simulink model "LaneMergingSim_ControllerWithVirtualHuman"  (R2015a)
settings: Solver=ode3  StartTime=0.0  StopTime=11.0  FixedStep=0.1  RelTol=1e-3
libraries: simulink x1
settings Model: Creator=ppnathan  LastModifiedBy=ppnathan

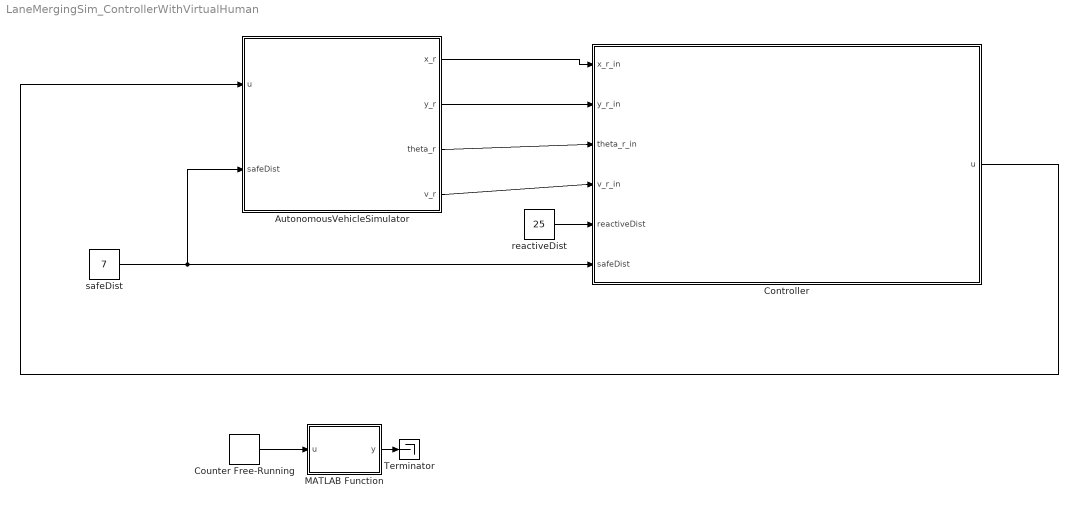
== system LaneMergingSim_ControllerWithVirtualHuman ==
  AutonomousVehicleSimulator : Subsystem
  Controller : Subsystem
  Counter Free-Running : simulink/Sources/Counter Free-Running  NumBits=32  tsamp=-1
  MATLAB Function : MATLAB Function  TreatAsAtomicUnit=on
  Terminator : Terminator
  reactiveDist : Constant  Value=25
  safeDist : Constant  Value=7
  wires:
  AutonomousVehicleSimulator/1(x_r) -> Controller/1(x_r_in)
  AutonomousVehicleSimulator/2(y_r) -> Controller/2(y_r_in)
  AutonomousVehicleSimulator/3(theta_r) -> Controller/3(theta_r_in)
  AutonomousVehicleSimulator/4(v_r) -> Controller/4(v_r_in)
  reactiveDist/1 -> Controller/5(reactiveDist)
  safeDist/1 -> AutonomousVehicleSimulator/2(safeDist), Controller/6(safeDist)
  Controller/1(u) -> AutonomousVehicleSimulator/1(u)
  Counter Free-Running/1 -> MATLAB Function/1(u)
  MATLAB Function/1(y) -> Terminator/1

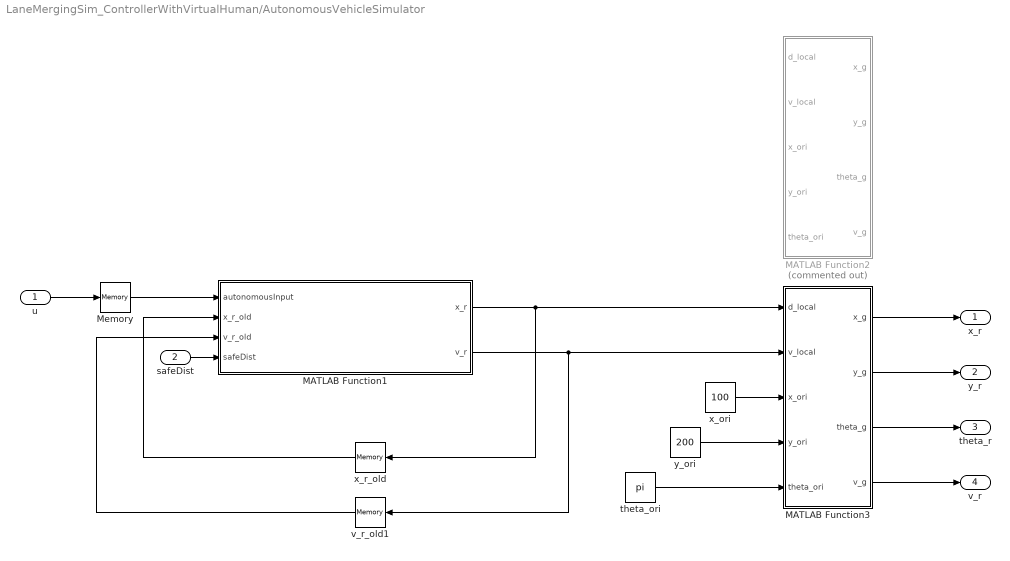
== system LaneMergingSim_ControllerWithVirtualHuman/AutonomousVehicleSimulator ==
  u : Inport
  safeDist : Inport  Port=2
  MATLAB Function1 : MATLAB Function  TreatAsAtomicUnit=on
  MATLAB Function2 : MATLAB Function  Commented=on  TreatAsAtomicUnit=on
  MATLAB Function3 : MATLAB Function  TreatAsAtomicUnit=on
  Memory : Memory
  theta_ori : Constant  Value=pi
  v_r_old1 : Memory  X0=31
  x_ori : Constant  Value=100
  x_r_old : Memory  X0=-330
  y_ori : Constant  Value=200
  x_r : Outport
  y_r : Outport  Port=2
  theta_r : Outport  Port=3
  v_r : Outport  Port=4
  wires:
  safeDist/1 -> MATLAB Function1/4(safeDist)
  MATLAB Function1/1(x_r) -> x_r_old/1, MATLAB Function3/1(d_local)
  MATLAB Function1/2(v_r) -> v_r_old1/1, MATLAB Function3/2(v_local)
  x_ori/1 -> MATLAB Function3/3(x_ori)
  y_ori/1 -> MATLAB Function3/4(y_ori)
  theta_ori/1 -> MATLAB Function3/5(theta_ori)
  MATLAB Function3/1(x_g) -> x_r/1
  MATLAB Function3/2(y_g) -> y_r/1
  MATLAB Function3/3(theta_g) -> theta_r/1
  MATLAB Function3/4(v_g) -> v_r/1
  u/1 -> Memory/1
  Memory/1 -> MATLAB Function1/1(autonomousInput)
  x_r_old/1 -> MATLAB Function1/2(x_r_old)
  v_r_old1/1 -> MATLAB Function1/3(v_r_old)

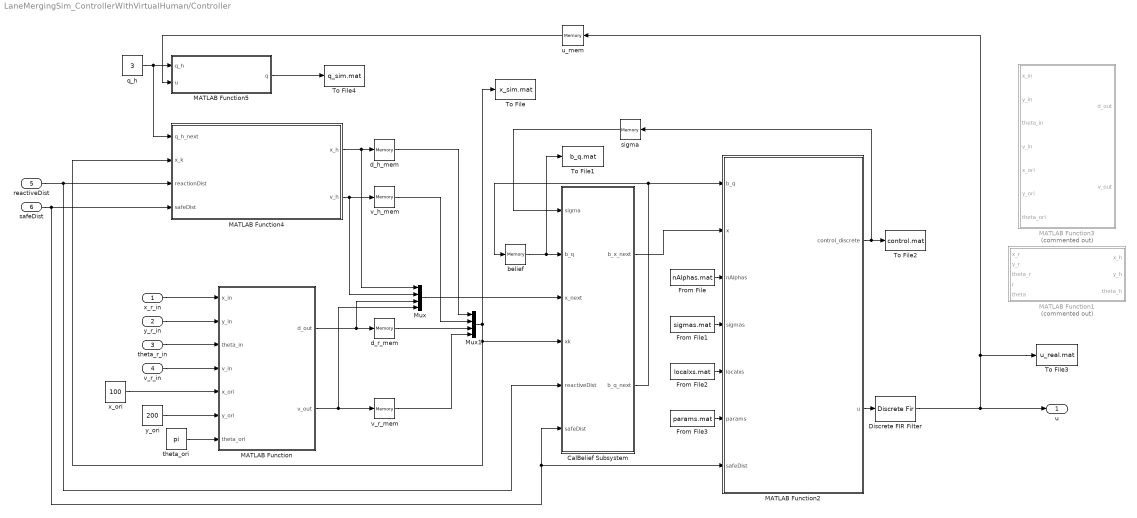
== system LaneMergingSim_ControllerWithVirtualHuman/Controller ==
  x_r_in : Inport
  y_r_in : Inport  Port=2
  theta_r_in : Inport  Port=3
  v_r_in : Inport  Port=4
  reactiveDist : Inport  Port=5
  safeDist : Inport  Port=6
  CalBelief Subsystem : Subsystem
  Discrete FIR Filter : DiscreteFir  Coefficients=[1/3 1/3 1/3]
  From File : FromFile  FileName=nAlphas.mat
  From File1 : FromFile  FileName=sigmas.mat
  From File2 : FromFile  FileName=localxs.mat
  From File3 : FromFile  FileName=params.mat
  MATLAB Function : MATLAB Function  TreatAsAtomicUnit=on
  MATLAB Function1 : MATLAB Function  Commented=on  TreatAsAtomicUnit=on
  MATLAB Function2 : MATLAB Function  TreatAsAtomicUnit=on
  MATLAB Function3 : MATLAB Function  Commented=on  TreatAsAtomicUnit=on
  MATLAB Function4 : MATLAB Function  TreatAsAtomicUnit=on
  MATLAB Function5 : MATLAB Function  TreatAsAtomicUnit=on
  Mux : Mux
  Mux1 : Mux
  To File : ToFile  Filename=x_sim.mat  MatrixName=x_sim
  To File1 : ToFile  Filename=b_q.mat  MatrixName=b_q
  To File2 : ToFile  Filename=control.mat  MatrixName=control
  To File3 : ToFile  Filename=u_real.mat  MatrixName=u_real
  To File4 : ToFile  Filename=q_sim.mat  MatrixName=q_sim
  belief : Memory  X0="[0.25, 0, 0, 0.25, 0, 0,  0.25, 0, 0, 0.25, 0, 0]"
  d_h_mem : Memory  X0=-300
  d_r_mem : Memory  X0=-330
  q_h : Constant  Value=3
  sigma : Memory  X0=1  InheritSampleTime=on
  theta_ori : Constant  Value=pi
  u_mem : Memory
  v_h_mem : Memory  X0=30
  v_r_mem : Memory  X0=31
  x_ori : Constant  Value=100
  y_ori : Constant  Value=200
  u : Outport
  wires:
  y_ori/1 -> MATLAB Function/6(y_ori)
  theta_ori/1 -> MATLAB Function/7(theta_ori)
  x_r_in/1 -> MATLAB Function/1(x_in)
  y_r_in/1 -> MATLAB Function/2(y_in)
  theta_r_in/1 -> MATLAB Function/3(theta_in)
  v_r_in/1 -> MATLAB Function/4(v_in)
  MATLAB Function/2(v_out) -> Mux/4, v_r_mem/1
  MATLAB Function/1(d_out) -> Mux/3, d_r_mem/1
  belief/1 -> To File1/1, CalBelief Subsystem/2(b_q)
  d_r_mem/1 -> Mux1/3
  v_r_mem/1 -> Mux1/4
  From File/1 -> MATLAB Function2/3(nAlphas)
  From File1/1 -> MATLAB Function2/4(sigmas)
  From File2/1 -> MATLAB Function2/5(localxs)
  From File3/1 -> MATLAB Function2/6(params)
  MATLAB Function2/1(control_discrete) -> To File2/1, sigma/1
  safeDist/1 -> MATLAB Function4/4(safeDist), CalBelief Subsystem/6(safeDist), MATLAB Function2/7(safeDist)
  x_ori/1 -> MATLAB Function/5(x_ori)
  d_h_mem/1 -> Mux1/1
  v_h_mem/1 -> Mux1/2
  Mux1/1 -> To File/1, MATLAB Function4/2(x_k), CalBelief Subsystem/4(xk)
  CalBelief Subsystem/1(b_x_next) -> MATLAB Function2/2(x)
  sigma/1 -> CalBelief Subsystem/1(sigma)
  Mux/1 -> CalBelief Subsystem/3(x_next)
  reactiveDist/1 -> MATLAB Function4/3(reactionDist), CalBelief Subsystem/5(reactiveDist)
  CalBelief Subsystem/2(b_q_next) -> MATLAB Function2/1(b_q), belief/1
  MATLAB Function2/2(u) -> Discrete FIR Filter/1
  Discrete FIR Filter/1 -> u_mem/1, To File3/1, u/1
  MATLAB Function4/1(x_h) -> Mux/1, d_h_mem/1
  MATLAB Function4/2(v_h) -> Mux/2, v_h_mem/1
  q_h/1 -> MATLAB Function4/1(q_h_next), MATLAB Function5/1(q_h)
  MATLAB Function5/1(q) -> To File4/1
  u_mem/1 -> MATLAB Function5/2(u)

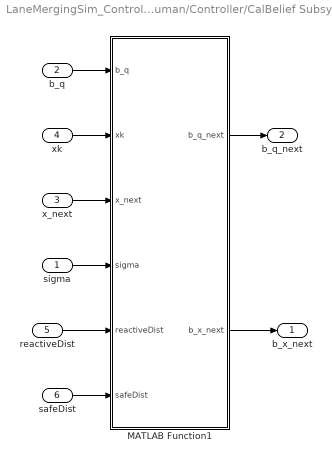
== system LaneMergingSim_ControllerWithVirtualHuman/Controller/CalBelief Subsystem ==
  sigma : Inport
  b_q : Inport  Port=2
  x_next : Inport  Port=3  PortDimensions=4
  xk : Inport  Port=4  PortDimensions=4
  reactiveDist : Inport  Port=5
  safeDist : Inport  Port=6
  MATLAB Function1 : MATLAB Function  TreatAsAtomicUnit=on
  b_x_next : Outport  PortDimensions=4
  b_q_next : Outport  Port=2  PortDimensions=12
  wires:
  reactiveDist/1 -> MATLAB Function1/5(reactiveDist)
  b_q/1 -> MATLAB Function1/1(b_q)
  xk/1 -> MATLAB Function1/2(xk)
  sigma/1 -> MATLAB Function1/4(sigma)
  MATLAB Function1/2(b_x_next) -> b_x_next/1
  safeDist/1 -> MATLAB Function1/6(safeDist)
  x_next/1 -> MATLAB Function1/3(x_next)
  MATLAB Function1/1(b_q_next) -> b_q_next/1

== matlab function LaneMergingSim_ControllerWithVirtualHuman/Controller/CalBelief Subsystem/MATLAB Function1 ==
  data: b_q input; b_q_next output; xk input; x_next input; sigma input; b_x_next output; reactiveDist input; safeDist input
function [b_q_next, b_x_next] = CalBelief(b_q, xk, x_next, sigma, reactiveDist, safeDist)

nDState = length(b_q);
b_q_next = zeros(nDState, 1);

if (norm(x_next - xk) < 1e-6)
    b_q_next = b_q;
else
    
    for qq = 1:nDState
        tmp = 0;
        for q = 1:nDState
            tmp = tmp + DStateTransfn(qq, q, sigma) * b_q(q);
        end
        b_q_next(qq) = DObsfn(0, qq) * ...
                       CStateTransfn(x_next, qq, xk, reactiveDist, safeDist) * tmp;
    end

    if (sum(b_q_next) == 0)
        b_q_next = b_q;
    else
        b_q_next = b_q_next / sum(b_q_next);
    end
end

b_x_next = x_next;

end

== matlab function LaneMergingSim_ControllerWithVirtualHuman/Controller/MATLAB Function ==
  data: x_in input; d_out output; y_in input; theta_in input; v_in input; x_ori input; y_ori input; theta_ori input; v_out output
function [d_out, v_out] = Global2Local(x_in, y_in, theta_in, v_in, x_ori, y_ori, theta_ori)

temp = [cos(-theta_ori) -sin(theta_ori);...
       sin(theta_ori) cos(theta_ori)] * [x_in - x_ori; y_in - y_ori];
x_local = temp(1);
theta_local = theta_in - theta_ori;

d_out = x_local;
v_out = v_in * cos(theta_local);

end

== matlab function LaneMergingSim_ControllerWithVirtualHuman/Controller/MATLAB Function2 ==
  data: b_q input; control_discrete output; x input; nAlphas input; sigmas input; localxs input; params input; safeDist input; u output
function [control_discrete, u] = FindOptimalContol(b_q, x, nAlphas, sigmas, localxs, params, safeDist)

nCState = length(x);
localxs = reshape(localxs, nCState, []);
params = reshape(params, 21, 12, []);
thresholddist = 10;
nDState = length(b_q);

bestvalue = -1e20;
bestidx = -1;

mindist = 1e20;
mindistidx = -1;

for n = 1:nAlphas
    sum  = 0;
    dist = norm(x - localxs(:, n));
    if (dist < thresholddist && (SatisfyConstraints(x, safeDist) || ...
		                         ~SatisfyConstraints(localxs(:, n), safeDist)))
        for q = 1:nDState
            const_term = params(1, q, n);
            first_order_term = params(2:(1+nCState), q, n);
            second_order_term = params((2+nCState):(1+nCState+nCState*nCState), q, n);
            second_order_term_reshape = reshape(second_order_term, nCState, nCState);
            sum = sum + b_q(q) * (const_term + first_order_term' * (x - localxs(:, n)) + ...
                                  (x - localxs(:, n))' * second_order_term_reshape * (x - localxs(:, n)));
        end
        
        if (sum > bestvalue)
            bestvalue = sum;
            bestidx = n;
        end
    end
    if (dist < mindist)
        mindist = dist;
        mindistidx = n;
    end
end

if (bestidx == -1)
    bestidx = mindistidx;
    disp('No point within the threshold, use policy with the nearest point.');
end

control_discrete = sigmas(bestidx);
disp('control_discrete = ');
disp(control_discrete);

if (control_discrete == 1) 
    u = 0;
elseif (control_discrete == 2)
    u = 1;
else
    u = -1;
end


end

== matlab function LaneMergingSim_ControllerWithVirtualHuman/AutonomousVehicleSimulator/MATLAB Function1 ==
  data: autonomousInput input; x_r output; x_r_old input; v_r_old input; safeDist input; v_r output
function [x_r, v_r] = SampleAutonomousVehicleState(autonomousInput, x_r_old, v_r_old, safeDist)

% if (~SatisfyConstraints(x_k, safeDist))
%     x_r =  x_k(3);
%     v_r =  x_k(4);
% else
    mNoiseMean = 0;
    mDistNoiseStd = 0.1;
    mVelNoiseStd = 0.1;
    mDeltaT = 0.1;
    
%     autonomousDriver = q_r_next;
%     
%     if (autonomousDriver == 1)
%         autonomousInput = 0;
%     elseif (autonomousDriver == 2)
%         autonomousInput = 1;
%     elseif (autonomousDriver == 3)
%         autonomousInput = -1;
%     else
%         autonomousInput = 0;
%         disp('SampleAutonomousVehicleState(): q_next out of domain');
%     end
    
    distNoise4AutonomousDriver = normrnd(mNoiseMean, mDistNoiseStd);
    velNoise4AutonomousDriver = normrnd(mNoiseMean, mVelNoiseStd);
    
    x_r = x_r_old + mDeltaT * v_r_old + distNoise4AutonomousDriver;
    v_r = v_r_old + mDeltaT * autonomousInput + velNoise4AutonomousDriver;
    
end

== matlab function LaneMergingSim_ControllerWithVirtualHuman/AutonomousVehicleSimulator/MATLAB Function2 ==
  data: d_local input; x_g output; v_local input; x_ori input; y_ori input; theta_ori input; y_g output; theta_g output; v_g output
function [x_g, y_g, theta_g, v_g] = Local2Global(d_local, v_local, x_ori, y_ori, theta_ori)

x_local = d_local;
y_local = 0;
temp = [cos(theta_ori) -sin(theta_ori); ...
        sin(theta_ori) cos(theta_ori)] * [x_local; y_local] + [x_ori; y_ori];

x_g = temp(1);
y_g = temp(2);
theta_g = theta_ori;

v_g = v_local;

end

== matlab function LaneMergingSim_ControllerWithVirtualHuman/Controller/MATLAB Function4 ==
  data: q_h_next input; x_h output; x_k input; reactionDist input; v_h output; safeDist input
function [x_h, v_h] = HumanDriverStateSimulator(q_h_next, x_k, reactionDist, safeDist)

if (~SatisfyConstraints(x_k, safeDist))
    x_h =  x_k(1);
    v_h =  x_k(2);
    
else
    OBLIVIOUS = 1; AGGRESSIVE = 2; COURTEOUS = 3; REASONABLE = 4;
    mNoiseMean = 0;
    mDistNoiseStd = 0.1;
    mVelNoiseStd = 0.1;
    mDeltaT = 0.1;

    humanDriver = q_h_next;

    if (humanDriver == OBLIVIOUS)
            humanInput = 0;
    elseif (humanDriver == AGGRESSIVE)
        if (abs(x_k(1) - x_k(3)) < reactionDist)
            humanInput = 1;
        else
            humanInput = 0;
        end
    elseif (humanDriver == COURTEOUS)
        if (abs(x_k(1) - x_k(3)) < reactionDist)
            humanInput = -1; 
        else
            humanInput = 0;
        end
    elseif (humanDriver == REASONABLE)
        if (abs(x_k(1) - x_k(3)) < reactionDist)
            if (x_k(2) > x_k(4))
                humanInput = 1;
            else
                humanInput = -1;
            end
        else
            humanInput = 0;
        end
    else
        humanInput = 0;
        disp('SampleHumanDriverState: q_next out of domain');
    end
    
    distNoise4HumanDriver = normrnd(mNoiseMean, mDistNoiseStd);
    velNoise4HumanDriver = normrnd(mNoiseMean, mVelNoiseStd);
    
    x_h = x_k(1) + mDeltaT * x_k(2) + distNoise4HumanDriver;
    v_h = x_k(2) + mDeltaT * humanInput + velNoise4HumanDriver;
end


end

== matlab function LaneMergingSim_ControllerWithVirtualHuman/AutonomousVehicleSimulator/MATLAB Function3 ==
  data: d_local input; x_g output; v_local input; x_ori input; y_ori input; theta_ori input; y_g output; theta_g output; v_g output
function [x_g, y_g, theta_g, v_g] = Local2Global(d_local, v_local, x_ori, y_ori, theta_ori)

x_local = d_local;
y_local = 0;
temp = [cos(theta_ori) -sin(theta_ori); ...
        sin(theta_ori) cos(theta_ori)] * [x_local; y_local] + [x_ori; y_ori];

x_g = temp(1);
y_g = temp(2);
theta_g = theta_ori;

v_g = v_local;

end

== matlab function LaneMergingSim_ControllerWithVirtualHuman/Controller/MATLAB Function3 ==
  data: x_in input; d_out output; y_in input; theta_in input; v_in input; x_ori input; y_ori input; theta_ori input; v_out output
function [d_out, v_out] = Global2Local(x_in, y_in, theta_in, v_in, x_ori, y_ori, theta_ori)


temp = [cos(-theta_ori) -sin(theta_ori);...
                      sin(theta_ori) cos(theta_ori)] * [x_in - x_ori; y_in - y_ori];
x_local = temp(1);
theta_local = theta_in - theta_ori;

d_out = x_local;
v_out = v_in * cos(theta_local);

end

== matlab function LaneMergingSim_ControllerWithVirtualHuman/MATLAB Function ==
  data: u input; y output
function y = PrintCounts(u)
disp('count = ');
disp(u);

y = u;

== matlab function LaneMergingSim_ControllerWithVirtualHuman/Controller/MATLAB Function5 ==
  data: q_h input; u input; q output
function q = Convert2DiscreteState(q_h, u)

if (u > 0)
    q_r  = 2;
elseif (u < 0)
    q_r = 3;
else
    q_r = 1;
end

q = (q_h - 1)*3 + q_r ;

end

== matlab function LaneMergingSim_ControllerWithVirtualHuman/Controller/MATLAB Function1 ==
  data: x_r input; x_h output; y_r input; theta_r input; r input; theta input; y_h output; theta_h output
function [x_h, y_h, theta_h] = Sensor2EgoLocal(x_r, y_r, theta_r, r, theta)

theta_h = theta_r;
x_h = x_r +cos(theta);
y_h = y_r + sin(theta);

end
